simulink model "DC_motor_model"  (R2016a)
settings: Solver=ode23tb  StartTime=0.0  StopTime=3  RelTol=1e-3
undefined symbols (not defined in the file or in its folder): B, J, Kb, Kt, L, R
settings Model: Creator=faiq1  LastModifiedBy=faiq1

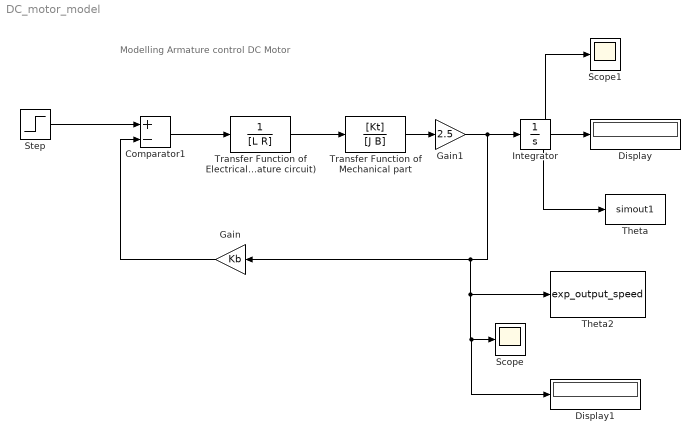
== system DC_motor_model ==
  note: Modelling Armature control DC Motor
  Comparator1 : Sum  Inputs=+-
  Display : Display
  Display1 : Display
  Gain : Gain  Gain=Kb
  Gain1 : Gain  Gain=2.5
  Integrator : Integrator
  Scope : Scope
  Scope1 : Scope
  Step : Step  Time=0  After=14.4  SampleTime=0
  Theta : ToWorkspace  VariableName=simout1  SaveFormat=Timeseries  SampleTime=-1
  Theta2 : ToWorkspace  VariableName=exp_output_speed  SaveFormat=Timeseries  SampleTime=-1
  Transfer Function of Electrical part (Armature circuit) : TransferFcn  Denominator=[L R]
  Transfer Function of Mechanical part : TransferFcn  Numerator=[Kt]  Denominator=[J B]
  wires:
  Transfer Function of Electrical part (Armature circuit)/1 -> Transfer Function of Mechanical part/1
  Integrator/1 -> Scope1/1, Display/1, Theta/1
  Step/1 -> Comparator1/1
  Gain/1 -> Comparator1/2
  Comparator1/1 -> Transfer Function of Electrical part (Armature circuit)/1
  Transfer Function of Mechanical part/1 -> Gain1/1
  Gain1/1 -> Display1/1, Scope/1, Theta2/1, Gain/1, Integrator/1
